simulink model "model"  (R2018a)
settings: Solver=FixedStepAuto  StartTime=0.0  StopTime=20  FixedStep=0.01  RelTol=1e-3
settings Model: EnablePacing=on  Creator=U500304  LastModifiedBy=U500304
settings SolverCC: ZeroCrossAlgorithm=Adaptive
settings DebuggingCC: MaxConsecutiveZCsMsg=none

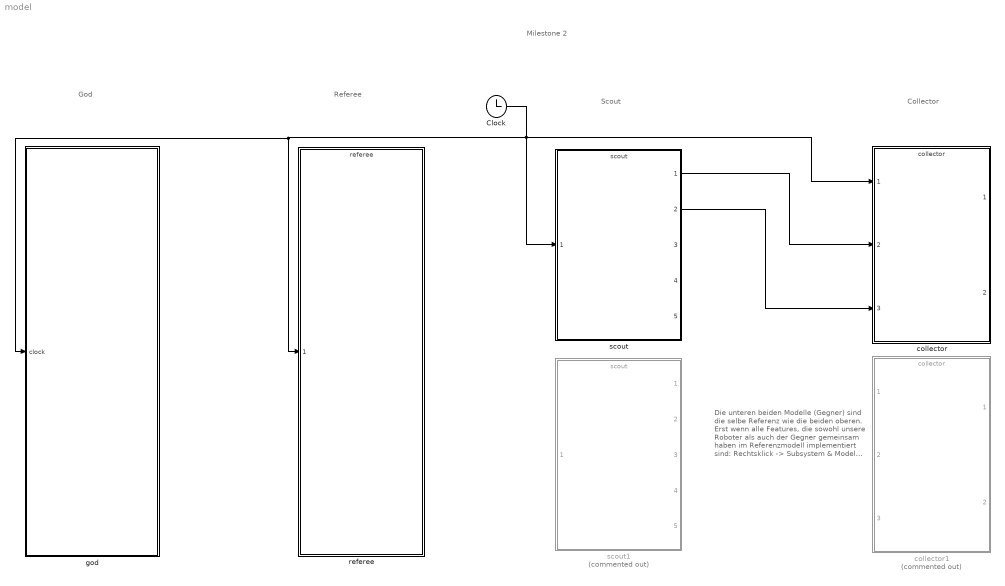
== system model ==
  note: Die unteren beiden Modelle (Gegner)
      | sind die selbe Referenz wie die beiden
      | oberen. Erst wenn alle Features, die
      | sowohl unsere Roboter als auch der
      | Gegner gemeinsam haben im
      | Referenzmodell implementiert sind:
      | Rechtsklick -> Subsystem & Model
      | Reference -> Convert to -> Variant Subsystem
  note: Milestone 2
  note: God
  note: Referee
  note: Scout
  note: Collector
  Clock : Clock
  collector : ModelReference  ModelNameDialog=collector  SimulationMode=Normal  ModelReferenceVersion=1.232
  collector1 : ModelReference  Commented=on  ModelNameDialog=collector  SimulationMode=Normal  ModelReferenceVersion=1.232
  god : Subsystem
  referee : ModelReference  ModelNameDialog=referee  SimulationMode=Normal  ModelReferenceVersion=1.239
  scout : ModelReference  ModelNameDialog=scout  SimulationMode=Normal  ModelReferenceVersion=1.229
  scout1 : ModelReference  Commented=on  ModelNameDialog=scout  SimulationMode=Normal  ModelReferenceVersion=1.229
  wires:
  Clock/1 -> god/1(clock), referee/1, scout/1, collector/1
  scout/1 -> collector/2
  scout/2 -> collector/3

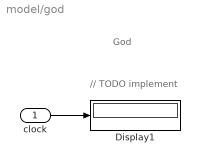
== system model/god ==
  note: // TODO implement
  note: God
  clock : Inport
  Display1 : Display
  wires:
  clock/1 -> Display1/1
